simulink model "csro_ctrl"  (R2021a)
settings: configuration reference "f2_sys_config" (kept outside this file)
values from neighbouring files (symbols this model uses):
  sys_regs = 1    [csro_ctrl_data.sldd]
libraries: simulink x1
settings Model: DataDictionary=csro_ctrl_data.sldd  Creator=Litao  LastModifiedBy=Litao
settings ConfigSetRef: SourceName=f2_sys_config

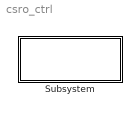
== system csro_ctrl ==
  Subsystem : Subsystem

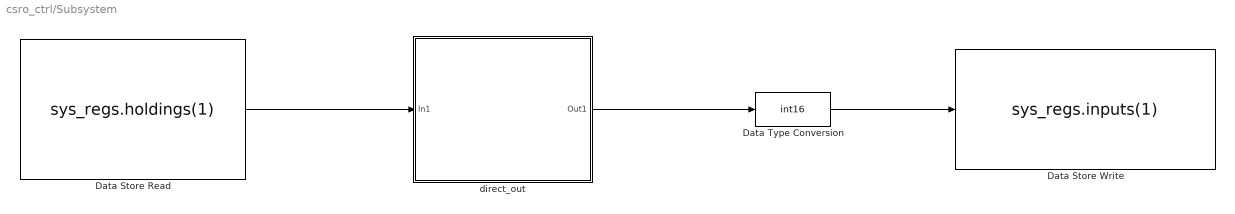
== system csro_ctrl/Subsystem ==
  Data Store Read : DataStoreRead  DataStoreName=sys_regs  DataStoreElements=sys_regs.holdings(1)  IndexOptions=Index vector (dialog)  Indices=1  OutputSizes=1
  Data Store Write : DataStoreWrite  DataStoreName=sys_regs  DataStoreElements=sys_regs.inputs(1)  IndexOptions=Index vector (dialog)  Indices=1  OutputSizes=1
  Data Type Conversion : DataTypeConversion  OutDataTypeStr=int16
  direct_out : Subsystem
  wires:
  Data Store Read/1 -> direct_out/1(In1)
  direct_out/1(Out1) -> Data Type Conversion/1
  Data Type Conversion/1 -> Data Store Write/1

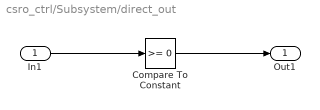
== system csro_ctrl/Subsystem/direct_out ==
  In1 : Inport
  Compare To Constant : simulink/Logic and Bit Operations/Compare To Constant  relop=>=  const=0  OutDataTypeStr=boolean
  Out1 : Outport
  wires:
  In1/1 -> Compare To Constant/1
  Compare To Constant/1 -> Out1/1
